simulink model "Isa_Lib"  (R2024b)
settings: Solver=VariableStepAuto  StartTime=0.0  StopTime=10.0  RelTol=1e-3

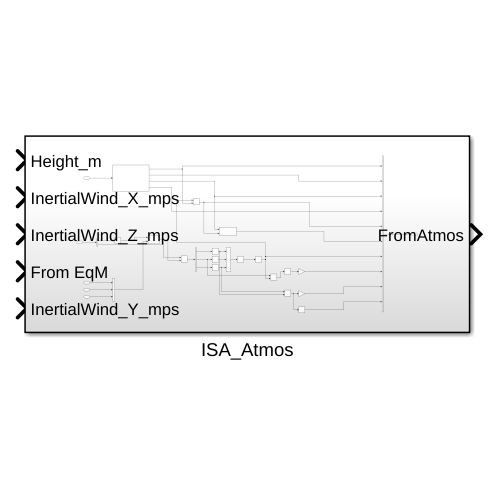
[thumbnail: Simulink's stored preview of the top-level diagram]
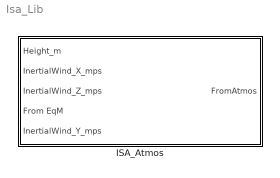
== system Isa_Lib ==
  ISA_Atmos : Subsystem

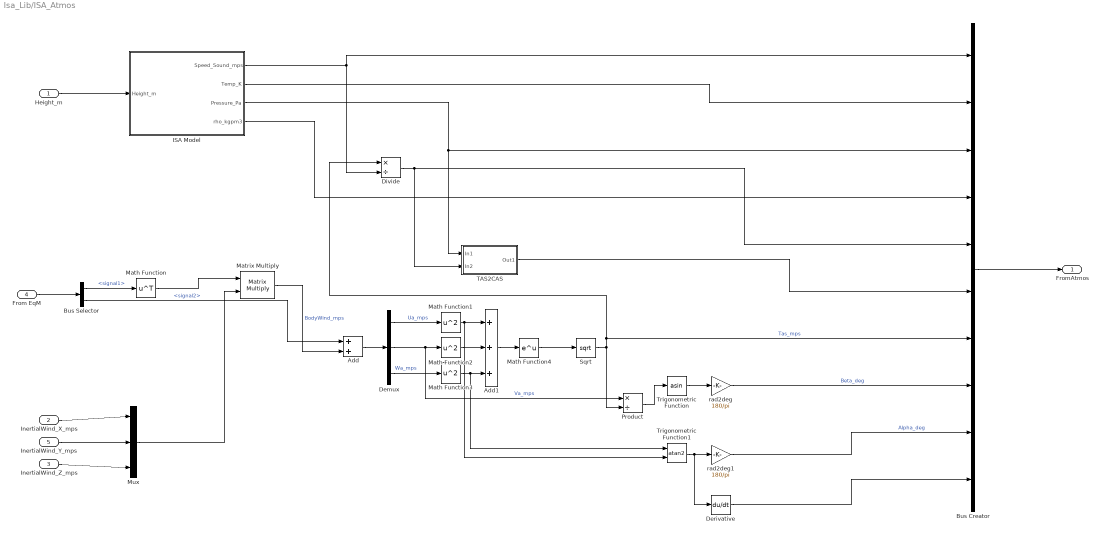
== system Isa_Lib/ISA_Atmos ==
  Height_m : Inport
  InertialWind_X_mps : Inport  Port=2
  InertialWind_Z_mps : Inport  Port=3
  From EqM : Inport  Port=4
  InertialWind_Y_mps : Inport  Port=5
  Add : Sum
  Add1 : Sum  Inputs=+++
  Bus Creator : BusCreator  Inputs=10
  Bus Selector : BusSelector  OutputSignals=signal1,signal2
  Demux : Demux  Outputs=3
  Derivative : Derivative
  Divide : Product  Inputs=*/
  ISA Model : Subsystem
  Math Function : Math  Operator=transpose
  Math Function1 : Math  Operator=square
  Math Function2 : Math  Operator=square
  Math Function3 : Math  Operator=square
  Math Function4 : Math
  Matrix Multiply : Product  Multiplication=Matrix(*)
  Mux : Mux  Inputs=3
  Product : Product  Inputs=*/
  Sqrt : Sqrt
  TAS2CAS : Subsystem
  Trigonometric Function : Trigonometry  Operator=asin
  Trigonometric Function1 : Trigonometry  Operator=atan2
  rad2deg : Gain  Gain=180/pi
  rad2deg1 : Gain  Gain=180/pi
  FromAtmos : Outport
  wires:
  Bus Selector/2 -> Add/1  "<signal2>"
  Math Function2/1 -> Add1/2
  rad2deg1/1 -> Bus Creator/9  "Alpha_deg"
  Product/1 -> Trigonometric Function/1
  InertialWind_X_mps/1 -> Mux/1
  Trigonometric Function/1 -> rad2deg/1
  Demux/2 -> Product/1, Math Function2/1  "Va_mps"
  Demux/3 -> Math Function3/1  "Wa_mps"
  ISA Model/2(Temp_K) -> Bus Creator/2
  Height_m/1 -> ISA Model/1(Height_m)
  Math Function1/1 -> Trigonometric Function1/2, Add1/1
  Sqrt/1 -> Bus Creator/7, Divide/1, Product/2  "Tas_mps"
  InertialWind_Y_mps/1 -> Mux/2
  ISA Model/1(Speed_Sound_mps) -> Divide/2, Bus Creator/1
  Math Function3/1 -> Trigonometric Function1/1, Add1/3
  ISA Model/3(Pressure_Pa) -> TAS2CAS/1(In1), Bus Creator/3
  Trigonometric Function1/1 -> Derivative/1, rad2deg1/1
  Math Function/1 -> Matrix Multiply/1
  Mux/1 -> Matrix Multiply/2
  InertialWind_Z_mps/1 -> Mux/3
  Bus Creator/1 -> FromAtmos/1
  Derivative/1 -> Bus Creator/10
  TAS2CAS/1(Out1) -> Bus Creator/6
  From EqM/1 -> Bus Selector/1
  ISA Model/4(rho_kgpm3) -> Bus Creator/4
  Demux/1 -> Math Function1/1  "Ua_mps"
  Bus Selector/1 -> Math Function/1  "<signal1>"
  rad2deg/1 -> Bus Creator/8  "Beta_deg"
  Add1/1 -> Math Function4/1
  Divide/1 -> Bus Creator/5, TAS2CAS/2(In2)
  Math Function4/1 -> Sqrt/1
  Add/1 -> Demux/1
  Matrix Multiply/1 -> Add/2  "BodyWind_mps"

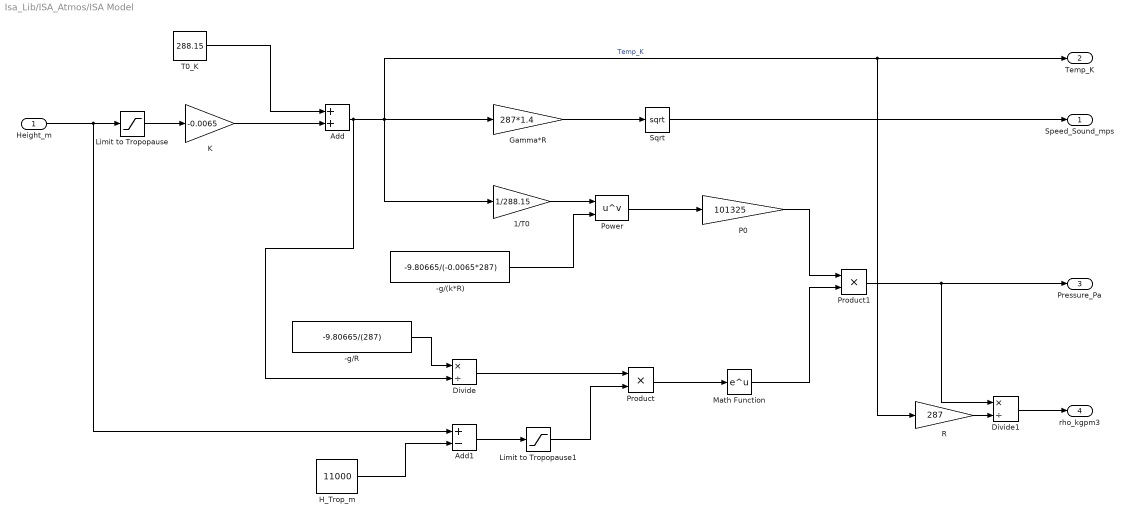
== system Isa_Lib/ISA_Atmos/ISA Model ==
  Height_m : Inport
  -g/(k*R) : Constant  Value=-9.80665/(-0.0065*287)
  -g/R : Constant  Value=-9.80665/(287)
  1/T0 : Gain  Gain=1/288.15
  Add : Sum
  Add1 : Sum  Inputs=+-
  Divide : Product  Inputs=*/
  Divide1 : Product  Inputs=*/
  Gamma*R : Gain  Gain=287*1.4
  H_Trop_m : Constant  Value=11000
  K : Gain  Gain=-0.0065
  Limit to Tropopause : Saturate  UpperLimit=11000  LowerLimit=0
  Limit to Tropopause1 : Saturate  UpperLimit=inf  LowerLimit=0
  Math Function : Math
  P0 : Gain  Gain=101325
  Power : Math  Operator=pow
  Product : Product
  Product1 : Product
  R : Gain  Gain=287
  Sqrt : Sqrt
  T0_K : Constant  Value=288.15
  Speed_Sound_mps : Outport
  Temp_K : Outport  Port=2
  Pressure_Pa : Outport  Port=3
  rho_kgpm3 : Outport  Port=4
  wires:
  T0_K/1 -> Add/1
  1/T0/1 -> Power/1
  -g/(k*R)/1 -> Power/2
  Limit to Tropopause/1 -> K/1
  -g/R/1 -> Divide/1
  Power/1 -> P0/1
  Height_m/1 -> Add1/1, Limit to Tropopause/1
  Sqrt/1 -> Speed_Sound_mps/1
  Add1/1 -> Limit to Tropopause1/1
  H_Trop_m/1 -> Add1/2
  Gamma*R/1 -> Sqrt/1
  Product1/1 -> Pressure_Pa/1, Divide1/1
  Limit to Tropopause1/1 -> Product/2
  Divide1/1 -> rho_kgpm3/1
  R/1 -> Divide1/2
  Add/1 -> R/1, Temp_K/1, 1/T0/1, Gamma*R/1, Divide/2  "Temp_K"
  K/1 -> Add/2
  P0/1 -> Product1/1
  Divide/1 -> Product/1
  Math Function/1 -> Product1/2
  Product/1 -> Math Function/1

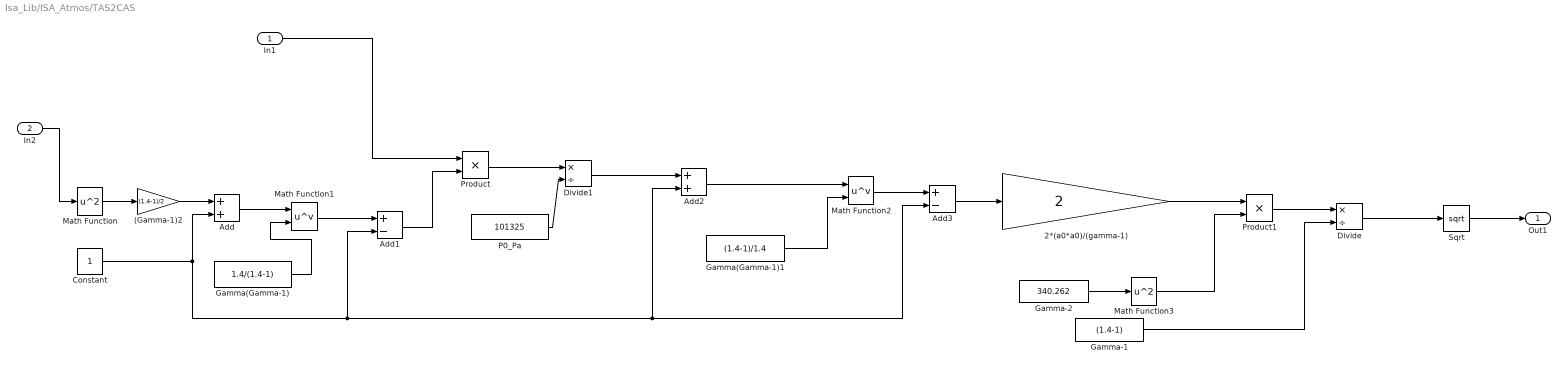
== system Isa_Lib/ISA_Atmos/TAS2CAS ==
  In1 : Inport
  In2 : Inport  Port=2
  (Gamma-1)2 : Gain  Gain=(1.4-1)/2
  2*(a0*a0)/(gamma-1) : Gain  Gain=2
  Add : Sum
  Add1 : Sum  Inputs=+-
  Add2 : Sum
  Add3 : Sum  Inputs=+-
  Constant : Constant
  Divide : Product  Inputs=*/
  Divide1 : Product  Inputs=*/
  Gamma(Gamma-1) : Constant  Value=1.4/(1.4-1)
  Gamma(Gamma-1)1 : Constant  Value=(1.4-1)/1.4
  Gamma-1 : Constant  Value=(1.4-1)
  Gamma-2 : Constant  Value=340.262
  Math Function : Math  Operator=square
  Math Function1 : Math  Operator=pow
  Math Function2 : Math  Operator=pow
  Math Function3 : Math  Operator=square
  P0_Pa : Constant  Value=101325
  Product : Product
  Product1 : Product
  Sqrt : Sqrt
  Out1 : Outport
  wires:
  Math Function/1 -> (Gamma-1)2/1
  (Gamma-1)2/1 -> Add/1
  Add1/1 -> Product/2
  Add/1 -> Math Function1/1
  In1/1 -> Product/1
  Gamma(Gamma-1)/1 -> Math Function1/2
  2*(a0*a0)/(gamma-1)/1 -> Product1/1
  P0_Pa/1 -> Divide1/2
  Add2/1 -> Math Function2/1
  Constant/1 -> Add1/2, Add2/2, Add3/2, Add/2
  Divide1/1 -> Add2/1
  Gamma(Gamma-1)1/1 -> Math Function2/2
  Math Function2/1 -> Add3/1
  Add3/1 -> 2*(a0*a0)/(gamma-1)/1
  Math Function1/1 -> Add1/1
  Sqrt/1 -> Out1/1
  Product/1 -> Divide1/1
  In2/1 -> Math Function/1
  Gamma-1/1 -> Divide/2
  Divide/1 -> Sqrt/1
  Gamma-2/1 -> Math Function3/1
  Math Function3/1 -> Product1/2
  Product1/1 -> Divide/1
